simulink model "ground_track_test"  (R2016b)
settings: Solver=VariableStepAuto  StartTime=0.0  StopTime=10800  RelTol=1e-3
undefined symbols (not defined in the file): fsw_params
libraries: GPS_time_lib x1, ground_visualization_lib x1, sgp4_lib_fsw x1, time_coord_rotation_lib x1
settings Model: Creator=Sean  LastModifiedBy=Sean

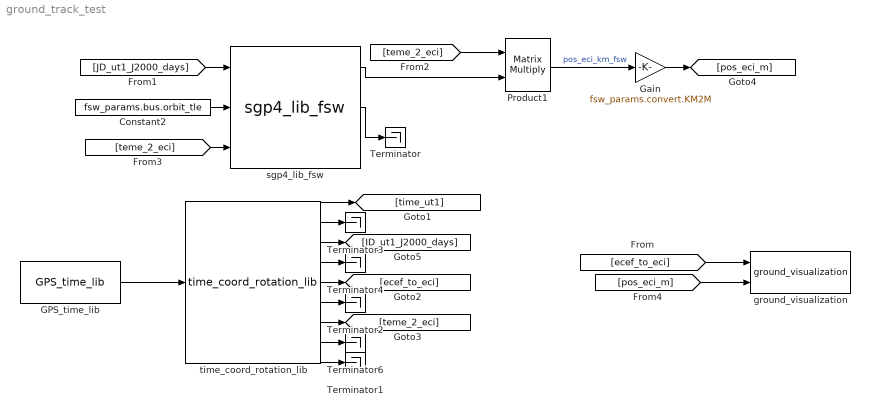
== system ground_track_test ==
  Constant2 : Constant  Value=fsw_params.bus.orbit_tle
  GPS_time_lib : GPS_time_lib/GPS_time_lib
  Gain : Gain  Gain=fsw_params.convert.KM2M
  Product1 : Product  Multiplication=Matrix(*)
  Terminator{,1..4,6} (6 alike) : Terminator
  ground_visualization : ground_visualization_lib/ground_visualization
  sgp4_lib_fsw : sgp4_lib_fsw/sgp4_lib_fsw
  time_coord_rotation_lib : time_coord_rotation_lib/time_coord_rotation_lib
  wires:
  time_coord_rotation_lib/8 -> Terminator6/1
  time_coord_rotation_lib/2 -> Terminator3/1
  time_coord_rotation_lib/1 -> [time_ut1]
  [ecef_to_eci] -> ground_visualization/1
  Gain/1 -> [pos_eci_m]
  Product1/1 -> Gain/1  "pos_eci_km_fsw"
  sgp4_lib_fsw/1 -> Product1/2
  [JD_ut1_J2000_days] -> sgp4_lib_fsw/1
  [teme_2_eci] -> Product1/1
  sgp4_lib_fsw/2 -> Terminator/1
  GPS_time_lib/1 -> time_coord_rotation_lib/1
  [pos_eci_m] -> ground_visualization/2
  Constant2/1 -> sgp4_lib_fsw/2
  [teme_2_eci] -> sgp4_lib_fsw/3
  time_coord_rotation_lib/5 -> [ecef_to_eci]
  time_coord_rotation_lib/7 -> [teme_2_eci]
  time_coord_rotation_lib/9 -> Terminator1/1
  time_coord_rotation_lib/6 -> Terminator2/1
  time_coord_rotation_lib/4 -> Terminator4/1
  time_coord_rotation_lib/3 -> [JD_ut1_J2000_days]
